simulink model "PubIfDecisionTOS_MDL"  (R2020b)
settings: configuration reference "DspaceConfig" (kept outside this file)
PostLoadFcn:
  | if any(exist('dsrtsu_mdlpostloadfcn', 'file') ~= 0), dsrtsu_mdlpostloadfcn('Execute', bdroot); end
InitFcn:
  | , if any(exist('dsmpb_private', 'file') ~= 0), dsmpb_private('dsmpb_mdlclblib', 'Init', bdroot); end,
undefined symbols (not defined in the file or in its folder): C_TOS_ACCEgoRAxletoFbumplength_m, C_TOS_ACCTargetFront_Flag, C_TOS_AEBJAPedObjDxThre_Val, C_TOS_AEBJAPedObjDyThre_Val, C_TOS_AEBJATargetSize_Val, C_TOS_AEBJAVehObjDxThre_Val, C_TOS_AEBJAVehObjDyThre_Val, C_TOS_AEBJuncPedTargetSize_Val, C_TOS_AEBLatObjDxThre_Val, C_TOS_AEBLatPedDyThre_Val, C_TOS_AEBLatTargetSize_Val, C_TOS_AEBLongTargetInEgoFront_Flag, C_TOS_axAbsGround_Parameter, C_TOS_CameraConfirmedFlag, C_TOS_CNsubjWidth, C_TOS_CurrentLaneCoreMinWidth_Val, C_TOS_CutInProb_Val_Zero, C_TOS_CutOutProb_Val_Zero, C_TOS_D2R_Val, C_TOS_DefaultValueObjectToCenterLine_dy, C_TOS_EgoCarWidth_Val, C_TOS_EgoDxRefPoint_m, C_TOS_EgoRAxletoFbumplength_m, C_TOS_HalfWidthVehicle_Con, C_TOS_HWA_CurrentLaneFlag, C_TOS_HWA_LeftLaneFlag, C_TOS_HWA_MovingDir_Vaild, C_TOS_HWA_MovState_Vaild, C_TOS_HWA_RightLaneFlag, C_TOS_LaneLineCourseErrorFront, C_TOS_LaneLineCourseErrorRear, C_TOS_MotorbikeDefaultWidth_m, C_TOS_NumberOfEffectiveTargets, C_TOS_Obj_Age_Val, C_TOS_Objdx_Constraint_Val, C_TOS_ObjectDefaultWidth_m, C_TOS_ObjInCurrentLane_Val, C_TOS_ObjInCurrentLaneValid, C_TOS_ObjInLeftLaneValid, C_TOS_ObjInRightLaneValid, C_TOS_ObjNotInCurrentLane_Val, C_TOS_ObjNotREElementType, C_TOS_ObjPredictDis_dy_ConstantVal_Zeros, C_TOS_ObjToCenterLine_ConstantVal_Zeros, C_TOS_OFMObjIDInvilad_Val, C_TOS_PIL_LatDisCons_Val_zero, C_TOS_PIL_ObjectCutInFlag_b, C_TOS_PIL_ObjectCutOutFlag_b, C_TOS_PIL_ObjLaneProb_al_Val, C_TOS_PP_ObjFusType_FC_Confirm_b, C_TOS_PP_ObjFusType_FC_FR_Confirm_b, C_TOS_PP_ObjFusType_FR_Confirm_b, C_TOS_RE_80BoolDefault_Val, C_TOS_RE_80Single181Default_Val, C_TOS_RE_80Single255Default_Val, C_TOS_RE_80Uint8Default_Val, C_TOS_RE_D2R, C_TOS_RE_D_180_Val, C_TOS_RE_InvalidObjectID_Val, C_TOS_RE_InvalidTargetChainDir_Val ... (+142)
libraries: simulink x1650, TOS_LIB x361, canfdmsglib x14
(part 21 of 69)

== system PubIfDecisionTOS_MDL/TOS_20201112/TOS_2012080320/TOS/AEB/TOS_AEBLatCro_20201208/AEBLat_Object_Condition/AEBLat_TargetCondition ==
  Object_ID : Inport  OutDataTypeStr=uint8  Partition=on  PartitionDimension=1  PartitionWidth=1  PartitionOffset=0
  PP_ObjFusType_FC_FR_Confirm : Inport  Port=2  Partition=on  PartitionDimension=1  PartitionWidth=1  PartitionOffset=0
  PP_ObjFusType_FR_Confirm : Inport  Port=3  Partition=on  PartitionDimension=1  PartitionWidth=1  PartitionOffset=0
  ObjectType : Inport  Port=4  Partition=on  PartitionDimension=1  PartitionWidth=1  PartitionOffset=0
  Object_Dx : Inport  Port=5  Partition=on  PartitionDimension=1  PartitionWidth=1  PartitionOffset=0
  Object_Dy : Inport  Port=6  Partition=on  PartitionDimension=1  PartitionWidth=1  PartitionOffset=0
  PP_ObjMovingDirSignalProcessing : Inport  Port=7  Partition=on  PartitionDimension=1  PartitionWidth=1  PartitionOffset=0
  Object_HeadingAngle : Inport  Port=8  Partition=on  PartitionDimension=1  PartitionWidth=1  PartitionOffset=0
  Object_VX : Inport  Port=9  Partition=on  PartitionDimension=1  PartitionWidth=1  PartitionOffset=0
  Object_VY : Inport  Port=10  Partition=on  PartitionDimension=1  PartitionWidth=1  PartitionOffset=0
  VIE_EgoVelocity : Inport  Port=11
  psiDtOpt : Inport  Port=12
  AEBLat_Target_ObjectID_K1 : Inport  Port=13
  Compare To Constant : simulink/Logic and Bit Operations/Compare To Constant  relop===  const=C_TOS_OFMObjIDInvilad_Val  OutDataTypeStr=boolean
      settings: AttributesFormatString=C_TOS_OFMObjIDInvilad_Val = 0
  For Each : ForEach  DisableCoverage=on
  If : If  IfExpression=u1 ~= 0
  Merge{,1..4} (5 alike) : Merge
  TOS_AEBLat_TargetsDx : Subsystem
  TOS_AEBLat_TargetsDxDefault : Subsystem  TreatAsAtomicUnit=on
  TOS_AEBLat_Targets_Dx : Outport  ConcatenationDimension=1
  AEBLat_TargetFusionType_observal : Outport  Port=2  ConcatenationDimension=1
  AEBLat_TargetObjectType_observal : Outport  Port=3  ConcatenationDimension=1
  AEBLat_TargetDXDY_observal : Outport  Port=4  ConcatenationDimension=1
  AEBLat_TargetMovDir_observal : Outport  Port=5  ConcatenationDimension=1
  wires:
  PP_ObjFusType_FC_FR_Confirm/1 -> TOS_AEBLat_TargetsDx/2(PP_ObjFusType_FC_FR_Confirm)
  PP_ObjFusType_FR_Confirm/1 -> TOS_AEBLat_TargetsDx/3(PP_ObjFusType_FR_Confirm)
  Object_VY/1 -> TOS_AEBLat_TargetsDx/10(Object_VY)
  VIE_EgoVelocity/1 -> TOS_AEBLat_TargetsDx/11(VIE_EgoVelocity)
  Object_VX/1 -> TOS_AEBLat_TargetsDx/9(Object_VX)
  PP_ObjMovingDirSignalProcessing/1 -> TOS_AEBLat_TargetsDx/7(PP_ObjMovingDirSignalProcessing)
  Object_HeadingAngle/1 -> TOS_AEBLat_TargetsDx/8(Object_HeadingAngle)
  ObjectType/1 -> TOS_AEBLat_TargetsDx/4(ObjectType)
  TOS_AEBLat_TargetsDxDefault/1(TOS_AEBLong_TargetsDx) -> Merge/1
  If/2 -> TOS_AEBLat_TargetsDx/Action
  If/1 -> TOS_AEBLat_TargetsDxDefault/Action
  Object_ID/1 -> Compare To Constant/1, [Object_ID]
  Compare To Constant/1 -> If/1
  TOS_AEBLat_TargetsDx/1(TOS_AEBLat_TargetsDx) -> Merge/2
  Object_Dy/1 -> TOS_AEBLat_TargetsDx/6(Object_Dy)
  Object_Dx/1 -> TOS_AEBLat_TargetsDx/5(Object_Dx)
  Merge/1 -> TOS_AEBLat_Targets_Dx/1
  TOS_AEBLat_TargetsDx/2(AEBLat_TargetFusionType_observal) -> Merge1/2
  TOS_AEBLat_TargetsDxDefault/2(AEBLong_TargetFusionType_observal) -> Merge1/1
  TOS_AEBLat_TargetsDxDefault/3(AEBLong_TargetObjectType_observal) -> Merge2/1
  TOS_AEBLat_TargetsDx/3(AEBLat_TargetObjectType_observal) -> Merge2/2
  TOS_AEBLat_TargetsDx/4(AEBLat_TargetDXDY_observal) -> Merge3/2
  TOS_AEBLat_TargetsDxDefault/4(AEBLong_TargetDXDY_observal) -> Merge3/1
  TOS_AEBLat_TargetsDxDefault/5(AEBLong_TargetMovDir_observal) -> Merge4/1
  TOS_AEBLat_TargetsDx/5(AEBLat_TargetMovDir_observal) -> Merge4/2
  Merge1/1 -> AEBLat_TargetFusionType_observal/1
  Merge2/1 -> AEBLat_TargetObjectType_observal/1
  Merge3/1 -> AEBLat_TargetDXDY_observal/1
  Merge4/1 -> AEBLat_TargetMovDir_observal/1
  [Object_ID] -> TOS_AEBLat_TargetsDx/1(Object_ID)  "Object_ID"
  AEBLat_Target_ObjectID_K1/1 -> TOS_AEBLat_TargetsDx/13(AEBLat_Target_ObjectID_K1)
  psiDtOpt/1 -> TOS_AEBLat_TargetsDx/12(psiDtOpt)

== system PubIfDecisionTOS_MDL/TOS_20201112/TOS_2012080320/TOS/AEB/TOS_AEBLatCro_20201208/AEBLat_Object_Condition2/AEBLat_TargetCondition ==
  Object_ID : Inport  OutDataTypeStr=uint8  Partition=on  PartitionDimension=1  PartitionWidth=1  PartitionOffset=0
  PP_ObjFusType_FC_FR_Confirm : Inport  Port=2  Partition=on  PartitionDimension=1  PartitionWidth=1  PartitionOffset=0
  PP_ObjFusType_FR_Confirm : Inport  Port=3  Partition=on  PartitionDimension=1  PartitionWidth=1  PartitionOffset=0
  ObjectType : Inport  Port=4  Partition=on  PartitionDimension=1  PartitionWidth=1  PartitionOffset=0
  Object_Dx : Inport  Port=5  Partition=on  PartitionDimension=1  PartitionWidth=1  PartitionOffset=0
  Object_Dy : Inport  Port=6  Partition=on  PartitionDimension=1  PartitionWidth=1  PartitionOffset=0
  PP_ObjMovingDirSignalProcessing : Inport  Port=7  Partition=on  PartitionDimension=1  PartitionWidth=1  PartitionOffset=0
  Object_HeadingAngle : Inport  Port=8  Partition=on  PartitionDimension=1  PartitionWidth=1  PartitionOffset=0
  Object_VX : Inport  Port=9  Partition=on  PartitionDimension=1  PartitionWidth=1  PartitionOffset=0
  Object_VY : Inport  Port=10  Partition=on  PartitionDimension=1  PartitionWidth=1  PartitionOffset=0
  VIE_EgoVelocity : Inport  Port=11
  psiDtOpt : Inport  Port=12
  AEBLat_Target_ObjectID_K1 : Inport  Port=13
  Compare To Constant : simulink/Logic and Bit Operations/Compare To Constant  relop===  const=C_TOS_OFMObjIDInvilad_Val  OutDataTypeStr=boolean
      settings: AttributesFormatString=C_TOS_OFMObjIDInvilad_Val = 0
  For Each : ForEach  DisableCoverage=on
  If : If  IfExpression=u1 ~= 0
  Merge{,1..4} (5 alike) : Merge
  TOS_AEBLat_TargetsDx : Subsystem
  TOS_AEBLat_TargetsDxDefault : Subsystem  TreatAsAtomicUnit=on
  TOS_AEBLat_Targets_Dx : Outport  ConcatenationDimension=1
  AEBLat_TargetFusionType_observal : Outport  Port=2  ConcatenationDimension=1
  AEBLat_TargetObjectType_observal : Outport  Port=3  ConcatenationDimension=1
  AEBLat_TargetDXDY_observal : Outport  Port=4  ConcatenationDimension=1
  AEBLat_TargetMovDir_observal : Outport  Port=5  ConcatenationDimension=1
  wires:
  PP_ObjFusType_FC_FR_Confirm/1 -> TOS_AEBLat_TargetsDx/2(PP_ObjFusType_FC_FR_Confirm)
  PP_ObjFusType_FR_Confirm/1 -> TOS_AEBLat_TargetsDx/3(PP_ObjFusType_FR_Confirm)
  Object_VY/1 -> TOS_AEBLat_TargetsDx/10(Object_VY)
  VIE_EgoVelocity/1 -> TOS_AEBLat_TargetsDx/11(VIE_EgoVelocity)
  Object_VX/1 -> TOS_AEBLat_TargetsDx/9(Object_VX)
  PP_ObjMovingDirSignalProcessing/1 -> TOS_AEBLat_TargetsDx/7(PP_ObjMovingDirSignalProcessing)
  Object_HeadingAngle/1 -> TOS_AEBLat_TargetsDx/8(Object_HeadingAngle)
  ObjectType/1 -> TOS_AEBLat_TargetsDx/4(ObjectType)
  TOS_AEBLat_TargetsDxDefault/1(TOS_AEBLong_TargetsDx) -> Merge/1
  If/2 -> TOS_AEBLat_TargetsDx/Action
  If/1 -> TOS_AEBLat_TargetsDxDefault/Action
  Object_ID/1 -> Compare To Constant/1, [Object_ID]
  Compare To Constant/1 -> If/1
  TOS_AEBLat_TargetsDx/1(TOS_AEBLat_TargetsDx) -> Merge/2
  Object_Dy/1 -> TOS_AEBLat_TargetsDx/6(Object_Dy)
  Object_Dx/1 -> TOS_AEBLat_TargetsDx/5(Object_Dx)
  Merge/1 -> TOS_AEBLat_Targets_Dx/1
  TOS_AEBLat_TargetsDx/2(AEBLat_TargetFusionType_observal) -> Merge1/2
  TOS_AEBLat_TargetsDxDefault/2(AEBLong_TargetFusionType_observal) -> Merge1/1
  TOS_AEBLat_TargetsDxDefault/3(AEBLong_TargetObjectType_observal) -> Merge2/1
  TOS_AEBLat_TargetsDx/3(AEBLat_TargetObjectType_observal) -> Merge2/2
  TOS_AEBLat_TargetsDx/4(AEBLat_TargetDXDY_observal) -> Merge3/2
  TOS_AEBLat_TargetsDxDefault/4(AEBLong_TargetDXDY_observal) -> Merge3/1
  TOS_AEBLat_TargetsDxDefault/5(AEBLong_TargetMovDir_observal) -> Merge4/1
  TOS_AEBLat_TargetsDx/5(AEBLat_TargetMovDir_observal) -> Merge4/2
  Merge1/1 -> AEBLat_TargetFusionType_observal/1
  Merge2/1 -> AEBLat_TargetObjectType_observal/1
  Merge3/1 -> AEBLat_TargetDXDY_observal/1
  Merge4/1 -> AEBLat_TargetMovDir_observal/1
  [Object_ID] -> TOS_AEBLat_TargetsDx/1(Object_ID)  "Object_ID"
  AEBLat_Target_ObjectID_K1/1 -> TOS_AEBLat_TargetsDx/13(AEBLat_Target_ObjectID_K1)
  psiDtOpt/1 -> TOS_AEBLat_TargetsDx/12(psiDtOpt)

== system PubIfDecisionTOS_MDL/TOS_20201112/TOS_2012080320/TOS/AEB/TOS_AEBLong/AEBLongTargetInfor/AEBLongTargetMovingDir ==
  TOS_AddAttributes : Inport
  TOS_AEBLongTargetIndex : Inport  Port=2  OutDataTypeStr=uint8
  AEBLongTargetInfroDefault : Subsystem  TreatAsAtomicUnit=on
  AEBLongTargetMovingDir : Subsystem  TreatAsAtomicUnit=on
  Compare To Constant1 : simulink/Logic and Bit Operations/Compare To Constant  relop===  const=C_TOS_OFMObjIDInvilad_Val  OutDataTypeStr=boolean
      settings: AttributesFormatString=C_TOS_OFMObjIDInvilad_Val = 0
  If : If  IfExpression=u1
  Merge : Merge
  TOS_AEBLongTargetMovingDir : Outport
  wires:
  Merge/1 -> TOS_AEBLongTargetMovingDir/1
  AEBLongTargetInfroDefault/1(TOS_AEBLongTargetMovingDir) -> Merge/1
  AEBLongTargetMovingDir/1(TOS_AEBLongTargetMovingDir) -> Merge/2
  If/2 -> AEBLongTargetMovingDir/Action
  If/1 -> AEBLongTargetInfroDefault/Action
  TOS_AddAttributes/1 -> AEBLongTargetMovingDir/1(TOS_AddAttributes)
  Compare To Constant1/1 -> If/1
  TOS_AEBLongTargetIndex/1 -> Compare To Constant1/1, AEBLongTargetMovingDir/2(TOS_AEBLongTargetIndex)

== system PubIfDecisionTOS_MDL/TOS_20201112/TOS_2012080320/TOS/AEB/TOS_AEBLong/AEBLong_Confirm/AEBLong ==
  Object_ID : Inport
  AEBLong_Index : Inport  Port=2
  Object_DX : Inport  Port=3
  Object_ObstacleProb : Inport  Port=4
  Object_ExistProb : Inport  Port=5
  Object_Fus_Type : Inport  Port=6
  object_MovingState : Inport  Port=7
  Object_HeadingAngle : Inport  Port=8
  Object_Type : Inport  Port=9
  VIE_EgoVelocity : Inport  Port=10
  PIL_LeftLaneProb : Inport  Port=11
  PIL_CurrentLaneProb : Inport  Port=12
  PIL_RightLaneProb : Inport  Port=13
  PP_MovingStateSignalProcessing : Inport  Port=14
  PP_ObjMovingDirSignalProcessing : Inport  Port=15
  PP_ObjectToCenterLine_dy : Inport  Port=16
  TLJ_TargetInCLValidityflg : Inport  Port=17
  PP_CurrentLaneWidth : Inport  Port=18
  Object_DY : Inport  Port=19
  SteerWheelAng : Inport  Port=20
  SteerWheelSpd : Inport  Port=21
  PP_ObjFusType_FC_FR_Confirm : Inport  Port=22
  PP_ObjFusType_FR_Confirm : Inport  Port=23
  PP_ObjFusType_FC_Confirm : Inport  Port=24
  Object_VX : Inport  Port=25
  Object_VY : Inport  Port=26
  PIL_OverlapRatio : Inport  Port=27
  AEBLong_Target_ID_K1 : Inport  Port=28
  AEBLong_Target_ID_K2 : Inport  Port=29
  AEBLong_Target_MovState_K1 : Inport  Port=30
  AEBLong_Target_MovState_K2 : Inport  Port=31
  AEBLong_TrgConfirm : Subsystem
  AEBLong_TrgConfirmDefault : Subsystem  TreatAsAtomicUnit=on
  Compare To Constant : simulink/Logic and Bit Operations/Compare To Constant  relop===  const=C_TOS_OFMObjIDInvilad_Val  OutDataTypeStr=boolean
      settings: AttributesFormatString=C_TOS_OFMObjIDInvilad_Val = 0
  Constant : Constant  Value=0  OutDataTypeStr=uint8
  If : If  IfExpression=u1 ~= 0
  Merge{,1..10} (11 alike) : Merge
  Switch : Switch  Criteria=u2 > Threshold
  TOS_AEBLong_TargetIndex : Outport
  TOS_AEBLong_TargetDis_ObserVale : Outport  Port=2
  TOS_AEBLong_ObstacleProb_ObserVale : Outport  Port=3
  TOS_AEBLong_TargetExistProb_ObserVale : Outport  Port=4
  TOS_AEBLong_ObjFusType_ObserVale : Outport  Port=5
  TOS_AEBLong_TargetInEgoFront_ObserVale : Outport  Port=6
  TOS_AEBLong_TargetMovingDir_ObserVale : Outport  Port=7
  TOS_AEB_Stockade_ObserVale : Outport  Port=8
  TOS_AEBLong_TargetDy_ObserVale : Outport  Port=9
  TOS_AEBLong_SteerWheelAngConfirm_ObserVale : Outport  Port=10
  TOS_AEBLong_OverlapRatio_ObserVale : Outport  Port=11
  wires:
  AEBLong_Index/1 -> [AEBLong_Index], Compare To Constant/1
  Merge/1 -> Switch/2
  Compare To Constant/1 -> If/1
  If/1 -> AEBLong_TrgConfirmDefault/Action
  AEBLong_TrgConfirmDefault/1(TOS_AEBLong_TargetConditionJudge) -> Merge/1
  Object_ID/1 -> AEBLong_TrgConfirm/2(Object_ID)
  Object_DX/1 -> AEBLong_TrgConfirm/3(Object_DX)
  Object_ObstacleProb/1 -> AEBLong_TrgConfirm/4(Object_ObstacleProb)
  Object_ExistProb/1 -> AEBLong_TrgConfirm/5(Object_ExistProb)
  Object_Fus_Type/1 -> AEBLong_TrgConfirm/6(Object_Fus_Type)
  object_MovingState/1 -> AEBLong_TrgConfirm/7(object_MovingState)
  Object_HeadingAngle/1 -> AEBLong_TrgConfirm/8(Object_HeadingAngle)
  Object_Type/1 -> AEBLong_TrgConfirm/9(Object_Type)
  VIE_EgoVelocity/1 -> AEBLong_TrgConfirm/10(VIE_EgoVelocity)
  PIL_LeftLaneProb/1 -> AEBLong_TrgConfirm/11(PIL_LeftLaneProb)
  PIL_CurrentLaneProb/1 -> AEBLong_TrgConfirm/12(PIL_CurrentLaneProb)
  PIL_RightLaneProb/1 -> AEBLong_TrgConfirm/13(PIL_RightLaneProb)
  PP_MovingStateSignalProcessing/1 -> AEBLong_TrgConfirm/14(PP_MovingStateSignalProcessing)
  PP_ObjMovingDirSignalProcessing/1 -> AEBLong_TrgConfirm/15(PP_ObjMovingDirSignalProcessing)
  PP_ObjectToCenterLine_dy/1 -> AEBLong_TrgConfirm/16(PP_ObjectToCenterLine_dy)
  TLJ_TargetInCLValidityflg/1 -> AEBLong_TrgConfirm/17(TLJ_TargetInCLValidityflg)
  PP_CurrentLaneWidth/1 -> AEBLong_TrgConfirm/18(PP_CurrentLaneWidth)
  Object_DY/1 -> AEBLong_TrgConfirm/19(Object_DY)
  SteerWheelAng/1 -> AEBLong_TrgConfirm/20(SteerWheelAng)  "SteerWheelAng"
  SteerWheelSpd/1 -> AEBLong_TrgConfirm/21(SteerWheelSpd)  "SteerWheelSpd"
  AEBLong_TrgConfirm/1(TOS_AEBLong_TargetConditionJudge) -> Merge/2
  If/2 -> AEBLong_TrgConfirm/Action
  [AEBLong_Index] -> AEBLong_TrgConfirm/1(In1)
  [AEBLong_Index] -> Switch/1
  Switch/1 -> TOS_AEBLong_TargetIndex/1
  Constant/1 -> Switch/3
  Merge7/1 -> TOS_AEBLong_TargetMovingDir_ObserVale/1
  Merge3/1 -> TOS_AEBLong_ObstacleProb_ObserVale/1
  Merge8/1 -> TOS_AEB_Stockade_ObserVale/1
  Merge10/1 -> TOS_AEBLong_SteerWheelAngConfirm_ObserVale/1
  Merge2/1 -> TOS_AEBLong_TargetDis_ObserVale/1
  Merge6/1 -> TOS_AEBLong_TargetInEgoFront_ObserVale/1
  Merge4/1 -> TOS_AEBLong_TargetExistProb_ObserVale/1
  Merge9/1 -> TOS_AEBLong_TargetDy_ObserVale/1
  Merge5/1 -> TOS_AEBLong_ObjFusType_ObserVale/1
  AEBLong_TrgConfirm/10(TOS_AEBLong_SteerWheelAngConfirm_ObserVale) -> Merge10/2
  AEBLong_TrgConfirm/2(TOS_AEBLong_TargetDis_ObserVale) -> Merge2/2
  AEBLong_TrgConfirm/3(TOS_AEBLong_ObstacleProb_ObserVale) -> Merge3/2
  AEBLong_TrgConfirm/4(TOS_AEBLong_TargetExistProb_ObserVale) -> Merge4/2
  AEBLong_TrgConfirm/5(TOS_AEBLong_ObjFusType_ObserVale) -> Merge5/2
  AEBLong_TrgConfirm/6(TOS_AEBLong_TargetInEgoFront_ObserVale) -> Merge6/2
  AEBLong_TrgConfirm/7(TOS_AEBLong_TargetMovingDir_ObserVale) -> Merge7/2
  AEBLong_TrgConfirm/8(TOS_AEB_Stockade_ObserVale) -> Merge8/2
  AEBLong_TrgConfirm/9(TOS_AEBLong_TargetDy_ObserVale) -> Merge9/2
  AEBLong_TrgConfirmDefault/2(TOS_AEBLong_TargetDis_ObserVale) -> Merge2/1
  AEBLong_TrgConfirmDefault/3(TOS_AEBLong_ObstacleProb_ObserVale) -> Merge3/1
  AEBLong_TrgConfirmDefault/4(TOS_AEBLong_TargetExistProb_ObserVale) -> Merge4/1
  AEBLong_TrgConfirmDefault/5(TOS_AEBLong_ObjFusType_ObserVale) -> Merge5/1
  AEBLong_TrgConfirmDefault/6(TOS_AEBLong_TargetInEgoFront_ObserVale) -> Merge6/1
  AEBLong_TrgConfirmDefault/7(TOS_AEBLong_TargetMovingDir_ObserVale) -> Merge7/1
  AEBLong_TrgConfirmDefault/8(TOS_AEB_Stockade_ObserVale) -> Merge8/1
  AEBLong_TrgConfirmDefault/9(TOS_AEBLong_TargetDy_ObserVale) -> Merge9/1
  AEBLong_TrgConfirmDefault/10(TOS_AEBLong_SteerWheelAngConfirm_ObserVale) -> Merge10/1
  PP_ObjFusType_FC_FR_Confirm/1 -> AEBLong_TrgConfirm/22(PP_ObjFusType_FC_FR_Confirm)
  PP_ObjFusType_FR_Confirm/1 -> AEBLong_TrgConfirm/23(PP_ObjFusType_FR_Confirm)
  PP_ObjFusType_FC_Confirm/1 -> AEBLong_TrgConfirm/24(PP_ObjFusType_FC_Confirm)
  Object_VX/1 -> AEBLong_TrgConfirm/25(Object_VX)
  Object_VY/1 -> AEBLong_TrgConfirm/26(Object_VY)
  PIL_OverlapRatio/1 -> AEBLong_TrgConfirm/27(PIL_OverlapRatio)
  AEBLong_TrgConfirmDefault/11(TOS_AEBLong_OverlapRatio_ObserVale) -> Merge1/1
  AEBLong_TrgConfirm/11(TOS_AEBLong_OverlapRatio_ObserVale) -> Merge1/2
  Merge1/1 -> TOS_AEBLong_OverlapRatio_ObserVale/1
  AEBLong_Target_ID_K1/1 -> AEBLong_TrgConfirm/28(AEBLong_Target_ID_K1)
  AEBLong_Target_ID_K2/1 -> AEBLong_TrgConfirm/29(AEBLong_Target_ID_K2)
  AEBLong_Target_MovState_K1/1 -> AEBLong_TrgConfirm/30(AEBLong_Target_MovState_K1)
  AEBLong_Target_MovState_K2/1 -> AEBLong_TrgConfirm/31(AEBLong_Target_MovState_K2)

== system PubIfDecisionTOS_MDL/TOS_20201112/TOS_2012080320/TOS/AEB/TOS_AEBLong/AEBLong_Confirm/TOS_AEBLong_ObserVale ==
  note: Obj_ID
  note: SteerWheelAngConfirm
  note: TargetDy
  note: Stockade
  note: TargetMovingDir
  note: TargetInEgoFront
  note: ObjFusType
  note: TargetExistProb
  note: ObstacleProb
  note: TargetDis
  TOS_AEBLong_TargetIndex : Inport
  TOS_AEBLong_ObserVale : Inport  Port=2
  Bus Selector3 : BusSelector  OutputSignals=TOS_AEBLong_TargetDis_ObserVale,TOS_AEBLong_ObstacleProb_ObserVale,TOS_AEBLong_TargetExistProb_ObserVale,TOS_AEBLong_ObjFusType_ObserVale,TOS_AEBLong_TargetInEgoFront_ObserVale,TOS_AEBLong_TargetMovingDir_ObserVale,TOS_AEB_Stockade_ObserVale,TOS_AEBLong_TargetDy_ObserVale,TOS_AEBLong_SteerWheelAngConfirm_ObserVale,TOS_AEBLong_OverlapRatio_ObserVale
  Display{,1..6,23..26} (11 alike) : Display
  wires:
  TOS_AEBLong_ObserVale/1 -> Bus Selector3/1
  Bus Selector3/1 -> [TOS_AEBLong_TargetDis_ObserVale]  "<TOS_AEBLong_TargetDis_ObserVale>"
  Bus Selector3/2 -> [TOS_AEBLong_ObstacleProb_ObserVale]  "<TOS_AEBLong_ObstacleProb_ObserVale>"
  Bus Selector3/3 -> [TOS_AEBLong_TargetExistProb_ObserVale]  "<TOS_AEBLong_TargetExistProb_ObserVale>"
  Bus Selector3/4 -> [TOS_AEBLong_ObjFusType_ObserVale]  "<TOS_AEBLong_ObjFusType_ObserVale>"
  Bus Selector3/5 -> [TOS_AEBLong_TargetInEgoFront_ObserVale]  "<TOS_AEBLong_TargetInEgoFront_ObserVale>"
  Bus Selector3/6 -> [TOS_AEBLong_TargetMovingDir_ObserVale]  "<TOS_AEBLong_TargetMovingDir_ObserVale>"
  Bus Selector3/7 -> [TOS_AEB_Stockade_ObserVale]  "<TOS_AEB_Stockade_ObserVale>"
  Bus Selector3/8 -> [TOS_AEB_TargetDy_ObserVale]  "<TOS_AEBLong_TargetDy_ObserVale>"
  Bus Selector3/9 -> [TOS_AEBLong_SteerWheelAngConfirm_ObserVale]  "<TOS_AEBLong_SteerWheelAngConfirm_ObserVale>"
  [TOS_AEBLong_TargetDis_ObserVale] -> Display26/1
  [TOS_AEBLong_ObstacleProb_ObserVale] -> Display25/1
  [TOS_AEBLong_TargetExistProb_ObserVale] -> Display24/1
  [TOS_AEBLong_ObjFusType_ObserVale] -> Display23/1
  [TOS_AEBLong_TargetInEgoFront_ObserVale] -> Display/1
  [TOS_AEBLong_TargetMovingDir_ObserVale] -> Display1/1
  [TOS_AEB_Stockade_ObserVale] -> Display2/1
  [TOS_AEB_TargetDy_ObserVale] -> Display3/1
  [TOS_AEBLong_SteerWheelAngConfirm_ObserVale] -> Display4/1
  TOS_AEBLong_TargetIndex/1 -> Display5/1
  Bus Selector3/10 -> [TOS_AEBLong_OverlapRatio_ObserVale]  "<TOS_AEBLong_OverlapRatio_ObserVale>"
  [TOS_AEBLong_OverlapRatio_ObserVale] -> Display6/1

== system PubIfDecisionTOS_MDL/TOS_20201112/TOS_2012080320/TOS/AEB/TOS_AEBLong/AEBLong_Target_PreJudge/AEBLONG_Target_PreFilt ==
  PP_ObjFusType_FC_FR_Confirm : Inport  Partition=on  PartitionDimension=1  PartitionWidth=1  PartitionOffset=0
  PP_ObjFusType_FR_Confirm : Inport  Port=2  Partition=on  PartitionDimension=1  PartitionWidth=1  PartitionOffset=0
  PP_ObjFusType_FC_Confirm : Inport  Port=3  Partition=on  PartitionDimension=1  PartitionWidth=1  PartitionOffset=0
  Object_ID : Inport  Port=4  OutDataTypeStr=uint8  Partition=on  PartitionDimension=1  PartitionWidth=1  PartitionOffset=0
  Obj_MovingState : Inport  Port=5  Partition=on  PartitionDimension=1  PartitionWidth=1  PartitionOffset=0
  Obj_Dx : Inport  Port=6  Partition=on  PartitionDimension=1  PartitionWidth=1  PartitionOffset=0
  Object_ObstacleProb : Inport  Port=7  Partition=on  PartitionDimension=1  PartitionWidth=1  PartitionOffset=0
  Object_DY : Inport  Port=8  Partition=on  PartitionDimension=1  PartitionWidth=1  PartitionOffset=0
  AEBLONG_Target_ID_K1 : Inport  Port=9
  AEBLONG_Target_Dx_K1 : Inport  Port=10
  PP_REElementType : Inport  Port=11  Partition=on  PartitionDimension=1  PartitionWidth=1  PartitionOffset=0
  AEBLONG_TargetPreCondJudge : Subsystem
  AEBLONG_TargetPreCondJudgeDefault : Subsystem  TreatAsAtomicUnit=on
  Compare To Constant : simulink/Logic and Bit Operations/Compare To Constant  relop===  const=C_TOS_OFMObjIDInvilad_Val  OutDataTypeStr=boolean
      settings: AttributesFormatString=C_TOS_OFMObjIDInvilad_Val = 0
  For Each : ForEach  DisableCoverage=on
  If : If  IfExpression=u1 ~= 0
  Merge{,1..4} (5 alike) : Merge
  TOS_AEBLONG_Target_PreFiltFlag : Outport  ConcatenationDimension=1
  TOS_AEBLONG_Target_FusionTypeFlag_ObserVale : Outport  Port=2  ConcatenationDimension=1
  TOS_AEBLONG_Target_PassedbyTarget_Flag_ObserVale : Outport  Port=3  ConcatenationDimension=1
  TOS_AEBLONG_Target_FenceFlag_ObserVale : Outport  Port=4  ConcatenationDimension=1
  TOS_AEBLONG_Target_REElementType_ObserVale : Outport  Port=5  ConcatenationDimension=1
  wires:
  Merge/1 -> TOS_AEBLONG_Target_PreFiltFlag/1
  PP_ObjFusType_FC_FR_Confirm/1 -> AEBLONG_TargetPreCondJudge/2(PP_ObjFusType_FC_FR_Confirm)
  PP_ObjFusType_FR_Confirm/1 -> AEBLONG_TargetPreCondJudge/3(PP_ObjFusType_FR_Confirm)
  AEBLONG_TargetPreCondJudge/1(TOS_AEBLONG_Target_PreFiltFlag) -> Merge/2
  Compare To Constant/1 -> If/1
  Object_ID/1 -> [Object_ID], Compare To Constant/1
  If/1 -> AEBLONG_TargetPreCondJudgeDefault/Action
  If/2 -> AEBLONG_TargetPreCondJudge/Action
  AEBLONG_TargetPreCondJudgeDefault/1(TOS_AEBLONG_Target_PreFiltFlag) -> Merge/1
  PP_ObjFusType_FC_Confirm/1 -> AEBLONG_TargetPreCondJudge/4(PP_ObjFusType_FC_Confirm)
  Obj_MovingState/1 -> AEBLONG_TargetPreCondJudge/5(Obj_MovingState)  "Obj_MovingState"
  Obj_Dx/1 -> AEBLONG_TargetPreCondJudge/6(Obj_Dx)  "Obj_Dx"
  Object_ObstacleProb/1 -> AEBLONG_TargetPreCondJudge/7(Object_ObstacleProb)  "Object_ObstacleProb"
  Object_DY/1 -> AEBLONG_TargetPreCondJudge/8(Object_DY)  "Object_DY"
  [Object_ID] -> AEBLONG_TargetPreCondJudge/1(Object_ID)
  AEBLONG_TargetPreCondJudge/2(TOS_AEBLONG_Target_FusionTypeFlag_ObserVale) -> Merge1/2
  AEBLONG_TargetPreCondJudge/3(TOS_AEBLONG_Target_PassedbyTarget_Flag_ObserVale) -> Merge2/2
  AEBLONG_TargetPreCondJudge/4(TOS_AEBLONG_Target_FenceFlag_ObserVale) -> Merge3/2
  AEBLONG_TargetPreCondJudgeDefault/2(TOS_AEBLONG_Target_FusionTypeFlag_ObserVale) -> Merge1/1
  AEBLONG_TargetPreCondJudgeDefault/3(TOS_AEBLONG_Target_PassedbyTarget_Flag_ObserVale) -> Merge2/1
  AEBLONG_TargetPreCondJudgeDefault/4(TOS_AEBLONG_Target_FenceFlag_ObserVale) -> Merge3/1
  Merge1/1 -> TOS_AEBLONG_Target_FusionTypeFlag_ObserVale/1
  Merge2/1 -> TOS_AEBLONG_Target_PassedbyTarget_Flag_ObserVale/1
  Merge3/1 -> TOS_AEBLONG_Target_FenceFlag_ObserVale/1
  AEBLONG_Target_ID_K1/1 -> AEBLONG_TargetPreCondJudge/9(AEBLONG_Target_ID_K1)  "AEBLONG_Target_ID_K1"
  AEBLONG_Target_Dx_K1/1 -> AEBLONG_TargetPreCondJudge/10(AEBLONG_Target_Dx_K1)  "AEBLONG_Target_Dx_K1"
  PP_REElementType/1 -> AEBLONG_TargetPreCondJudge/11(PP_REElementType)  "PP_REElementType"
  AEBLONG_TargetPreCondJudge/5(TOS_AEBLONG_Target_REElementType_ObserVale) -> Merge4/2
  AEBLONG_TargetPreCondJudgeDefault/5(TOS_AEBLONG_Target_REElementType_ObserVale) -> Merge4/1
  Merge4/1 -> TOS_AEBLONG_Target_REElementType_ObserVale/1

== system PubIfDecisionTOS_MDL/TOS_20201112/TOS_2012080320/TOS/LC_LCKie_ELK/TOS_HWA/CurrentLane/HWA_CurrentLane_Target ==
  note: 本车道前方，最近目标
  note: 前方次近
  VIE_EgoVelocity : Inport
  OFM_SignalVerification : Inport  Port=2
  TOS_AddAttributes : Inport  Port=3
  TOS_TLJ_SameLaneConfirm_Flag : Inport  Port=4
  TOS_ProbInLaneCalculat : Inport  Port=5
  TOS_VCAN_SignalVerification : Inport  Port=6
  LM_LR_Line04_dDisStart : Inport  Port=7
  LM_LR_Line04_dDisEnd : Inport  Port=8
  LM_LR_Line05_dDisStart : Inport  Port=9
  LM_LR_Line05_dDisEnd : Inport  Port=10
  LM_LR_Line06_dDisStart : Inport  Port=11
  LM_LR_Line06_dDisEnd : Inport  Port=12
  LM_LR_Line04_pC2 : Inport  Port=13
  LM_LR_Line05_pC2 : Inport  Port=14
  LM_LR_Line06_pC2 : Inport  Port=15
  LM_LR_Line04_fCamValid : Inport  Port=16
  LM_LR_Line05_fCamValid : Inport  Port=17
  LM_LR_Line06_fCamValid : Inport  Port=18
  LM_LR_Line04_pC0 : Inport  Port=19
  LM_RL_Line04_pC0 : Inport  Port=20
  TOS_HWA_Target_ID_K1 : Inport  Port=21
  TOS_HWA_Target_MovState_K1 : Inport  Port=22
  TOS_HWA_CurrentLane_ObjIndex : Inport  Port=23
  Bus Creator : BusCreator  Inputs=29
  Bus Creator1 : BusCreator  Inputs=18
  Bus Creator2 : BusCreator  Inputs=18
  Bus Creator3 : BusCreator  Inputs=5
  Bus Selector : BusSelector  OutputSignals=TOS_HWA_CurrentLane_ObjIndex,OFM_SignalVerification.Object_ID,OFM_SignalVerification.Object_Fus_Type,OFM_SignalVerification.Object_MovingState,TOS_AddAttributes.PP_ObjMovingDirSignalProcessing,OFM_SignalVerification.Object_HeadingAngle,OFM_SignalVerification.Object_DX,TOS_TLJ_SameLaneConfirm_Flag,OFM_SignalVerification.Object_Type,OFM_SignalVerification.Object_ObstacleProb,OFM_SignalVerification.Object_DY,TOS_AddAttributes.PP_ObjFusType_FC_FR_Confirm,TOS_AddAttributes.PP_ObjFusType_FR_Confirm,TOS_AddAttributes.PP_ObjFusType_FC_Confirm,OFM_SignalVerification.Object_VX,OFM_SignalVerification.Object_VY,VIE_EgoVelocity,TOS_VCAN_SignalVerification.SteerWheelAng,TOS_ProbInLaneCalculat.PIL_OverlapRatio,HWA_CLF_Target_2_ID_K1,HWA_CLF_Target_2_ID_K2,HWA_CLF_Target_2_MovState_K1,HWA_CLF_Target_2_MovState_K2,LM_LR_Line04_dDisStart,LM_LR_Line04_dDisEnd,LM_LR_Line05_dDisStart,LM_LR_Line05_dDisEnd,LM_LR_Line06_dDisStart,LM_LR_Line06_dDisEnd,LM_LR_Line04_pC2,LM_LR_Line05_pC2,LM_LR_Line06_pC2,LM_LR_Line04_fCamValid,LM_LR_Line05_fCamValid,LM_LR_Line06_fCamValid,LM_LR_Line04_pC0,LM_RL_Line04_pC0
  Bus Selector1 : BusSelector  OutputSignals=TOS_HWA_CurrentLane_ObjIndex,OFM_SignalVerification.Object_ID,OFM_SignalVerification.Object_Fus_Type,OFM_SignalVerification.Object_MovingState,TOS_AddAttributes.PP_ObjMovingDirSignalProcessing,OFM_SignalVerification.Object_HeadingAngle,OFM_SignalVerification.Object_DX,TOS_TLJ_SameLaneConfirm_Flag,OFM_SignalVerification.Object_Type,OFM_SignalVerification.Object_ObstacleProb,OFM_SignalVerification.Object_DY,TOS_AddAttributes.PP_ObjFusType_FC_FR_Confirm,TOS_AddAttributes.PP_ObjFusType_FR_Confirm,TOS_AddAttributes.PP_ObjFusType_FC_Confirm,OFM_SignalVerification.Object_VX,OFM_SignalVerification.Object_VY,VIE_EgoVelocity,TOS_VCAN_SignalVerification.SteerWheelAng,TOS_ProbInLaneCalculat.PIL_OverlapRatio,HWA_CLF_Target_1_ID_K1,HWA_CLF_Target_1_ID_K2,HWA_CLF_Target_1_MovState_K1,HWA_CLF_Target_1_MovState_K2,LM_LR_Line04_dDisStart,LM_LR_Line04_dDisEnd,LM_LR_Line05_dDisStart,LM_LR_Line05_dDisEnd,LM_LR_Line06_dDisStart,LM_LR_Line06_dDisEnd,LM_LR_Line04_pC2,LM_LR_Line05_pC2,LM_LR_Line06_pC2,LM_LR_Line04_fCamValid,LM_LR_Line05_fCamValid,LM_LR_Line06_fCamValid,LM_LR_Line04_pC0,LM_RL_Line04_pC0
  Bus Selector2 : BusSelector  OutputSignals=TOS_HWA_CurrentLane_ObjIndex,TOS_AddAttributes.PP_ObjMovingDirSignalProcessing,OFM_SignalVerification.Object_VX,OFM_SignalVerification.Object_VY,OFM_SignalVerification.Object_Type,OFM_SignalVerification.Object_MovingState,TOS_TLJ_SameLaneConfirm_Flag,OFM_SignalVerification.Object_DX,OFM_SignalVerification.Object_DY,OFM_SignalVerification.Object_Fus_Type,OFM_SignalVerification.Object_HeadingAngle,TOS_AddAttributes.PP_ObjFusType_FC_FR_Confirm,TOS_AddAttributes.PP_ObjFusType_FR_Confirm,TOS_AddAttributes.PP_ObjFusType_FC_Confirm,VIE_EgoVelocity
  Constant : Constant  Value=10  OutDataTypeStr=uint8
  Constant1 : Constant  Value=9  OutDataTypeStr=uint8
  Data Type Conversion{1..4} (4 alike) : DataTypeConversion  OutDataTypeStr=Enum: ObjectMovingState_E
  Delay{,3..4,7} (4 alike) : Delay  InitialCondition=0
  Delay{1..2,5..6} (4 alike) : Delay  DelayLength=1  InitialCondition=0
  HWA_CLF_Target_1 : Subsystem
  HWA_CLF_Target_2 : Subsystem
  HWA_CLF_Target_3 : Subsystem
  Selector{1..4} (4 alike) : Selector  InputPortWidth=11  IndexOptions=Index vector (port)  Indices=[1 3]  OutputSizes=1
  Subsystem : Subsystem
  TOS_HWA_Target_ID_K2 : InportShadow  Port=21
  TOS_HWA_Target_MovState_K2 : InportShadow  Port=22
  Terminator : Terminator
  Terminator1 : Terminator
  Terminator2 : Terminator
  HWA_CLF_Target_1_Index : Outport
  HWA_CLF_Target_2_Index : Outport  Port=2
  HWA_CLR_Target_3_Index : Outport  Port=3
  TargetInCurrentLane_b : Outport  Port=4
  wires:
  TOS_TLJ_SameLaneConfirm_Flag/1 -> Bus Creator/4  "TOS_TLJ_SameLaneConfirm_Flag"
  TOS_AddAttributes/1 -> Bus Creator/3  "TOS_AddAttributes"
  OFM_SignalVerification/1 -> Bus Creator/2  "OFM_SignalVerification"
  VIE_EgoVelocity/1 -> Bus Creator/1  "VIE_EgoVelocity"
  TOS_ProbInLaneCalculat/1 -> Bus Creator/5  "TOS_ProbInLaneCalculat"
  Bus Selector/3 -> HWA_CLF_Target_2/3(Object_Fus_Type)  "<Object_Fus_Type>"
  Bus Selector/4 -> HWA_CLF_Target_2/4(object_MovingState)  "<Object_MovingState>"
  HWA_CLF_Target_2/1(HWA_CLF_Target_2_Index) -> [HWA_CLF_Target_2_Index], HWA_CLF_Target_2_Index/1  "HWA_CLF_Target_2_Index"
  Bus Selector/7 -> HWA_CLF_Target_2/7(Object_DX)  "<Object_DX>"
  Bus Selector/8 -> HWA_CLF_Target_2/8(TOS_TLJ_SameLaneConfirm_Flag)  "<TOS_TLJ_SameLaneConfirm_Flag>"
  Bus Selector/9 -> HWA_CLF_Target_2/9(Object_Type)  "<Object_Type>"
  Bus Selector/2 -> HWA_CLF_Target_2/2(Object_ID)  "<Object_ID>"
  HWA_CLF_Target_2/2(HWA_CLF_Target_FusionType_ObserVale) -> Bus Creator1/1  "HWA_CLF_Target_2_FusionType_ObserVale"
  HWA_CLF_Target_2/3(HWA_CLF_Target_TrgMovDir_ObserVale) -> Bus Creator1/2  "HWA_CLF_Target_2_TrgMovDir_ObserVale"
  HWA_CLF_Target_2/4(HWA_CLF_Target_TargetDxConfirm_ObserVale) -> Bus Creator1/3  "HWA_CLF_Target_2_TargetDxConfirm_ObserVale"
  HWA_CLF_Target_2/5(HWA_CLF_Target_ObjType_ObserVale) -> Bus Creator1/4  "HWA_CLF_Target_2_ObjType_ObserVale"
  Bus Selector/10 -> HWA_CLF_Target_2/10(Object_ObstacleProb)  "<Object_ObstacleProb>"
  HWA_CLF_Target_2/6(HWA_CLF_Target_ObstacleProb_ObserVale) -> Bus Creator1/5  "HWA_CLF_Target_2_ObstacleProb_ObserVale"
  Bus Selector/5 -> HWA_CLF_Target_2/5(PP_ObjMovingDirSignalProcessing)  "<PP_ObjMovingDirSignalProcessing>"
  Bus Selector/6 -> HWA_CLF_Target_2/6(Object_HeadingAngle)  "<Object_HeadingAngle>"
  Bus Selector/11 -> HWA_CLF_Target_2/11(Object_DY)  "<Object_DY>"
  HWA_CLF_Target_2/7(HWA_CLF_Target_DyConfirm_ObserVale) -> Bus Creator1/6  "HWA_CLF_Target_2_DyConfirm_ObserVale"
  Bus Creator1/1 -> Terminator/1  "HWA_CLF_Target_2_ObserVale"
  TOS_HWA_CurrentLane_ObjIndex/1 -> Bus Creator/21  "TOS_HWA_CurrentLane_ObjIndex"
  Bus Selector/1 -> HWA_CLF_Target_2/1(HWA_CLF_Trg_2_Index)  "<TOS_HWA_CurrentLane_ObjIndex>"
  Bus Selector/12 -> HWA_CLF_Target_2/12(PP_ObjFusType_FC_FR_Confirm)  "<PP_ObjFusType_FC_FR_Confirm>"
  Bus Selector/13 -> HWA_CLF_Target_2/13(PP_ObjFusType_FR_Confirm)  "<PP_ObjFusType_FR_Confirm>"
  Bus Selector/14 -> HWA_CLF_Target_2/14(PP_ObjFusType_FC_Confirm)  "<PP_ObjFusType_FC_Confirm>"
  Bus Selector/15 -> HWA_CLF_Target_2/15(Object_VX)  "<Object_VX>"
  Bus Selector/16 -> HWA_CLF_Target_2/16(Object_VY)  "<Object_VY>"
  Bus Selector/17 -> HWA_CLF_Target_2/17(VIE_EgoVelocity)  "<VIE_EgoVelocity>"
  TOS_VCAN_SignalVerification/1 -> Bus Creator/6  "TOS_VCAN_SignalVerification"
  Bus Selector/18 -> HWA_CLF_Target_2/18(SteerWheelAng)  "<SteerWheelAng>"
  Bus Selector/19 -> HWA_CLF_Target_2/19(PIL_OverlapRatio)  "<PIL_OverlapRatio>"
  HWA_CLF_Target_2/17(HWA_CLF_Target_DyConfirm_4_OverlapRatio_ObserVale) -> Bus Creator1/16  "HWA_CLF_Target_2_DyConfirm_4_OverlapRatio_ObserVale"
  Delay1/1 -> Bus Creator/22  "HWA_CLF_Target_2_ID_K1"
  Delay/1 -> Bus Creator/23  "HWA_CLF_Target_2_ID_K2"
  Delay2/1 -> Data Type Conversion2/1
  Data Type Conversion1/1 -> Bus Creator/25  "HWA_CLF_Target_2_MovState_K2"
  Bus Selector/20 -> HWA_CLF_Target_2/20(HWA_CLF_Target_ID_K1)  "<HWA_CLF_Target_2_ID_K1>"
  Bus Selector/21 -> HWA_CLF_Target_2/21(HWA_CLF_Target_ID_K2)  "<HWA_CLF_Target_2_ID_K2>"
  Bus Selector/22 -> HWA_CLF_Target_2/22(HWA_CLF_Target_MovState_K1)  "<HWA_CLF_Target_2_MovState_K1>"
  Bus Selector/23 -> HWA_CLF_Target_2/23(HWA_CLF_Target_MovState_K2)  "<HWA_CLF_Target_2_MovState_K2>"
  Selector2/1 -> Delay3/1, Delay2/1
  Data Type Conversion2/1 -> Bus Creator/24  "HWA_CLF_Target_2_MovState_K1"
  HWA_CLF_Target_2/8(HWA_CLF_Target_TrgMovDirFlag_1_ObserVale) -> Bus Creator1/7  "HWA_CLF_Target_2_TrgMovDirFlag_1_ObserVale"
  HWA_CLF_Target_2/9(HWA_CLF_Target_TrgMovDirFlag_2_ObserVale) -> Bus Creator1/8  "HWA_CLF_Target_2_TrgMovDirFlag_2_ObserVale"
  HWA_CLF_Target_2/10(HWA_CLF_Target_TrgMovDirFlag_3_ObserVale) -> Bus Creator1/9  "HWA_CLF_Target_2_TrgMovDirFlag_3_ObserVale"
  HWA_CLF_Target_2/11(HWA_CLF_Target_TrgMovDirFlag_4_ObserVale) -> Bus Creator1/10  "HWA_CLF_Target_2_TrgMovDirFlag_4_ObserVale"
  HWA_CLF_Target_2/12(HWA_CLF_Target_TrgMovDirFlag_5_ObserVale) -> Bus Creator1/11  "HWA_CLF_Target_2_TrgMovDirFlag_5_ObserVale"
  HWA_CLF_Target_2/14(HWA_CLF_Target_DyConfirm_1_ObserVale) -> Bus Creator1/13  "HWA_CLF_Target_2_DyConfirm_1_ObserVale"
  HWA_CLF_Target_2/15(HWA_CLF_Target_DyConfirm_2_ObserVale) -> Bus Creator1/14  "HWA_CLF_Target_2_DyConfirm_2_ObserVale"
  HWA_CLF_Target_2/16(HWA_CLF_Target_DyConfirm_3_ObserVale) -> Bus Creator1/15  "HWA_CLF_Target_2_DyConfirm_3_ObserVale"
  Delay3/1 -> Data Type Conversion1/1
  TOS_HWA_Target_ID_K1/1 -> Selector1/1
  Selector3/1 -> Delay4/1, Delay5/1
  Selector4/1 -> Delay7/1, Delay6/1
  Delay5/1 -> Bus Creator/26  "HWA_CLF_Target_1_ID_K1"
  Delay4/1 -> Bus Creator/27  "HWA_CLF_Target_1_ID_K2"
  Delay6/1 -> Data Type Conversion4/1
  Delay7/1 -> Data Type Conversion3/1
  Data Type Conversion3/1 -> Bus Creator/29  "HWA_CLF_Target_1_MovState_K2"
  Data Type Conversion4/1 -> Bus Creator/28  "HWA_CLF_Target_1_MovState_K1"
  HWA_CLF_Target_2/13(HWA_CLF_Target_TrgMovDirFlag_6_ObserVale) -> Bus Creator1/12  "HWA_CLF_Target_2_TrgMovDirFlag_6_ObserVale"
  LM_LR_Line04_dDisStart/1 -> Bus Creator/7  "LM_LR_Line04_dDisStart"
  LM_LR_Line04_dDisEnd/1 -> Bus Creator/8  "LM_LR_Line04_dDisEnd"
  LM_LR_Line05_dDisStart/1 -> Bus Creator/9  "LM_LR_Line05_dDisStart"
  LM_LR_Line05_dDisEnd/1 -> Bus Creator/10  "LM_LR_Line05_dDisEnd"
  LM_LR_Line06_dDisStart/1 -> Bus Creator/11  "LM_LR_Line06_dDisStart"
  LM_LR_Line06_dDisEnd/1 -> Bus Creator/12  "LM_LR_Line06_dDisEnd"
  LM_LR_Line04_pC2/1 -> Bus Creator/13  "LM_LR_Line04_pC2"
  LM_LR_Line05_pC2/1 -> Bus Creator/14  "LM_LR_Line05_pC2"
  LM_LR_Line06_pC2/1 -> Bus Creator/15  "LM_LR_Line06_pC2"
  Bus Selector/24 -> HWA_CLF_Target_2/24(LM_LR_Line04_dDisStart)  "<LM_LR_Line04_dDisStart>"
  Bus Selector/25 -> HWA_CLF_Target_2/25(LM_LR_Line04_dDisEnd)  "<LM_LR_Line04_dDisEnd>"
  Bus Selector/26 -> HWA_CLF_Target_2/26(LM_LR_Line05_dDisStart)  "<LM_LR_Line05_dDisStart>"
  Bus Selector/27 -> HWA_CLF_Target_2/27(LM_LR_Line05_dDisEnd)  "<LM_LR_Line05_dDisEnd>"
  Bus Selector/28 -> HWA_CLF_Target_2/28(LM_LR_Line06_dDisStart)  "<LM_LR_Line06_dDisStart>"
  Bus Selector/29 -> HWA_CLF_Target_2/29(LM_LR_Line06_dDisEnd)  "<LM_LR_Line06_dDisEnd>"
  Bus Selector/30 -> HWA_CLF_Target_2/30(LM_LR_Line04_pC2)  "<LM_LR_Line04_pC2>"
  Bus Selector/31 -> HWA_CLF_Target_2/31(LM_LR_Line05_pC2)  "<LM_LR_Line05_pC2>"
  Bus Selector/32 -> HWA_CLF_Target_2/32(LM_LR_Line06_pC2)  "<LM_LR_Line06_pC2>"
  LM_LR_Line04_fCamValid/1 -> Bus Creator/16  "LM_LR_Line04_fCamValid"
  LM_LR_Line05_fCamValid/1 -> Bus Creator/17  "LM_LR_Line05_fCamValid"
  LM_LR_Line06_fCamValid/1 -> Bus Creator/18  "LM_LR_Line06_fCamValid"
  Bus Selector/33 -> HWA_CLF_Target_2/33(LM_LR_Line04_fCamValid)  "<LM_LR_Line04_fCamValid>"
  Bus Selector/34 -> HWA_CLF_Target_2/34(LM_LR_Line05_fCamValid)  "<LM_LR_Line05_fCamValid>"
  Bus Selector/35 -> HWA_CLF_Target_2/35(LM_LR_Line06_fCamValid)  "<LM_LR_Line06_fCamValid>"
  HWA_CLF_Target_2/18(HWA_CLF_Target_DyConfirm_5_OverlapConfirm_ObserVale) -> Bus Creator1/17  "HWA_CLF_Target_2_DyConfirm_5_OverlapConfirm_ObserVale"
  HWA_CLF_Target_2/19(HWA_CLF_Target_DyConfirm_ALL_6_ObserVale) -> Bus Creator1/18  "HWA_CLF_Target_2_DyConfirm_ALL_6_ObserVale"
  LM_LR_Line04_pC0/1 -> Bus Creator/19  "LM_LR_Line04_pC0"
  LM_RL_Line04_pC0/1 -> Bus Creator/20  "LM_RL_Line04_pC0"
  Bus Selector/36 -> HWA_CLF_Target_2/36(LM_LR_Line04_pC0)  "<LM_LR_Line04_pC0>"
  Bus Selector/37 -> HWA_CLF_Target_2/37(LM_RL_Line04_pC0)  "<LM_RL_Line04_pC0>"
  Selector1/1 -> Delay/1, Delay1/1
  Constant1/1 -> Selector4/2, Selector3/2
  Constant/1 -> Selector1/2, Selector2/2
  TOS_HWA_Target_MovState_K1/1 -> Selector2/1
  TOS_HWA_Target_ID_K2/1 -> Selector3/1
  TOS_HWA_Target_MovState_K2/1 -> Selector4/1
  Bus Selector1/37 -> HWA_CLF_Target_1/37(LM_RL_Line04_pC0)  "<LM_RL_Line04_pC0>"
  Bus Selector1/36 -> HWA_CLF_Target_1/36(LM_LR_Line04_pC0)  "<LM_LR_Line04_pC0>"
  HWA_CLF_Target_1/19(HWA_CLF_Target_DyConfirm_ALL_6_ObserVale) -> Bus Creator2/18  "HWA_CLF_Target_1_DyConfirm_ALL_6_ObserVale"
  HWA_CLF_Target_1/18(HWA_CLF_Target_DyConfirm_5_OverlapConfirm_ObserVale) -> Bus Creator2/17  "HWA_CLF_Target_1_DyConfirm_5_OverlapConfirm_ObserVale"
  Bus Selector1/35 -> HWA_CLF_Target_1/35(LM_LR_Line06_fCamValid)  "<LM_LR_Line06_fCamValid>"
  Bus Selector1/34 -> HWA_CLF_Target_1/34(LM_LR_Line05_fCamValid)  "<LM_LR_Line05_fCamValid>"
  Bus Selector1/33 -> HWA_CLF_Target_1/33(LM_LR_Line04_fCamValid)  "<LM_LR_Line04_fCamValid>"
  Bus Selector1/32 -> HWA_CLF_Target_1/32(LM_LR_Line06_pC2)  "<LM_LR_Line06_pC2>"
  Bus Selector1/31 -> HWA_CLF_Target_1/31(LM_LR_Line05_pC2)  "<LM_LR_Line05_pC2>"
  Bus Selector1/30 -> HWA_CLF_Target_1/30(LM_LR_Line04_pC2)  "<LM_LR_Line04_pC2>"
  Bus Selector1/29 -> HWA_CLF_Target_1/29(LM_LR_Line06_dDisEnd)  "<LM_LR_Line06_dDisEnd>"
  Bus Selector1/28 -> HWA_CLF_Target_1/28(LM_LR_Line06_dDisStart)  "<LM_LR_Line06_dDisStart>"
  Bus Selector1/27 -> HWA_CLF_Target_1/27(LM_LR_Line05_dDisEnd)  "<LM_LR_Line05_dDisEnd>"
  Bus Selector1/26 -> HWA_CLF_Target_1/26(LM_LR_Line05_dDisStart)  "<LM_LR_Line05_dDisStart>"
  Bus Selector1/25 -> HWA_CLF_Target_1/25(LM_LR_Line04_dDisEnd)  "<LM_LR_Line04_dDisEnd>"
  Bus Selector1/24 -> HWA_CLF_Target_1/24(LM_LR_Line04_dDisStart)  "<LM_LR_Line04_dDisStart>"
  HWA_CLF_Target_1/13(HWA_CLF_Target_TrgMovDirFlag_6_ObserVale) -> Bus Creator2/12  "HWA_CLF_Target_1_TrgMovDirFlag_6_ObserVale"
  HWA_CLF_Target_1/16(HWA_CLF_Target_DyConfirm_3_ObserVale) -> Bus Creator2/15  "HWA_CLF_Target_1_DyConfirm_3_ObserVale"
  HWA_CLF_Target_1/15(HWA_CLF_Target_DyConfirm_2_ObserVale) -> Bus Creator2/14  "HWA_CLF_Target_1_DyConfirm_2_ObserVale"
  HWA_CLF_Target_1/14(HWA_CLF_Target_DyConfirm_1_ObserVale) -> Bus Creator2/13  "HWA_CLF_Target_1_DyConfirm_1_ObserVale"
  HWA_CLF_Target_1/12(HWA_CLF_Target_TrgMovDirFlag_5_ObserVale) -> Bus Creator2/11  "HWA_CLF_Target_1_TrgMovDirFlag_5_ObserVale"
  HWA_CLF_Target_1/11(HWA_CLF_Target_TrgMovDirFlag_4_ObserVale) -> Bus Creator2/10  "HWA_CLF_Target_1_TrgMovDirFlag_4_ObserVale"
  HWA_CLF_Target_1/10(HWA_CLF_Target_TrgMovDirFlag_3_ObserVale) -> Bus Creator2/9  "HWA_CLF_Target_1_TrgMovDirFlag_3_ObserVale"
  HWA_CLF_Target_1/9(HWA_CLF_Target_TrgMovDirFlag_2_ObserVale) -> Bus Creator2/8  "HWA_CLF_Target_1_TrgMovDirFlag_2_ObserVale"
  HWA_CLF_Target_1/8(HWA_CLF_Target_TrgMovDirFlag_1_ObserVale) -> Bus Creator2/7  "HWA_CLF_Target_1_TrgMovDirFlag_1_ObserVale"
  Bus Selector1/23 -> HWA_CLF_Target_1/23(HWA_CLF_Target_MovState_K2)  "<HWA_CLF_Target_1_MovState_K2>"
  Bus Selector1/22 -> HWA_CLF_Target_1/22(HWA_CLF_Target_MovState_K1)  "<HWA_CLF_Target_1_MovState_K1>"
  Bus Selector1/21 -> HWA_CLF_Target_1/21(HWA_CLF_Target_ID_K2)  "<HWA_CLF_Target_1_ID_K2>"
  Bus Selector1/20 -> HWA_CLF_Target_1/20(HWA_CLF_Target_ID_K1)  "<HWA_CLF_Target_1_ID_K1>"
  HWA_CLF_Target_1/17(HWA_CLF_Target_DyConfirm_4_OverlapRatio_ObserVale) -> Bus Creator2/16  "HWA_CLF_Target_1_DyConfirm_4_OverlapRatio_ObserVale"
  Bus Selector1/19 -> HWA_CLF_Target_1/19(PIL_OverlapRatio)  "<PIL_OverlapRatio>"
  Bus Selector1/18 -> HWA_CLF_Target_1/18(SteerWheelAng)  "<SteerWheelAng>"
  Bus Selector1/17 -> HWA_CLF_Target_1/17(VIE_EgoVelocity)  "<VIE_EgoVelocity>"
  Bus Selector1/16 -> HWA_CLF_Target_1/16(Object_VY)  "<Object_VY>"
  Bus Selector1/15 -> HWA_CLF_Target_1/15(Object_VX)  "<Object_VX>"
  Bus Selector1/14 -> HWA_CLF_Target_1/14(PP_ObjFusType_FC_Confirm)  "<PP_ObjFusType_FC_Confirm>"
  Bus Selector1/13 -> HWA_CLF_Target_1/13(PP_ObjFusType_FR_Confirm)  "<PP_ObjFusType_FR_Confirm>"
  Bus Selector1/12 -> HWA_CLF_Target_1/12(PP_ObjFusType_FC_FR_Confirm)  "<PP_ObjFusType_FC_FR_Confirm>"
  Bus Selector1/1 -> HWA_CLF_Target_1/1(HWA_CLF_Trg_1_Index)  "<TOS_HWA_CurrentLane_ObjIndex>"
  Bus Creator2/1 -> Terminator1/1  "HWA_CLF_Target_1_ObserVale"
  HWA_CLF_Target_1/7(HWA_CLF_Target_DyConfirm_ObserVale) -> Bus Creator2/6  "HWA_CLF_Target_1_DyConfirm_ObserVale"
  Bus Selector1/11 -> HWA_CLF_Target_1/11(Object_DY)  "<Object_DY>"
  Bus Selector1/6 -> HWA_CLF_Target_1/6(Object_HeadingAngle)  "<Object_HeadingAngle>"
  Bus Selector1/5 -> HWA_CLF_Target_1/5(PP_ObjMovingDirSignalProcessing)  "<PP_ObjMovingDirSignalProcessing>"
  HWA_CLF_Target_1/6(HWA_CLF_Target_ObstacleProb_ObserVale) -> Bus Creator2/5  "HWA_CLF_Target_1_ObstacleProb_ObserVale"
  Bus Selector1/10 -> HWA_CLF_Target_1/10(Object_ObstacleProb)  "<Object_ObstacleProb>"
  HWA_CLF_Target_1/5(HWA_CLF_Target_ObjType_ObserVale) -> Bus Creator2/4  "HWA_CLF_Target_1_ObjType_ObserVale"
  HWA_CLF_Target_1/4(HWA_CLF_Target_TargetDxConfirm_ObserVale) -> Bus Creator2/3  "HWA_CLF_Target_1_TargetDxConfirm_ObserVale"
  HWA_CLF_Target_1/3(HWA_CLF_Target_TrgMovDir_ObserVale) -> Bus Creator2/2  "HWA_CLF_Target_1_TrgMovDir_ObserVale"
  HWA_CLF_Target_1/2(HWA_CLF_Target_FusionType_ObserVale) -> Bus Creator2/1  "HWA_CLF_Target_1_FusionType_ObserVale"
  Bus Selector1/2 -> HWA_CLF_Target_1/2(Object_ID)  "<Object_ID>"
  Bus Selector1/9 -> HWA_CLF_Target_1/9(Object_Type)  "<Object_Type>"
  Bus Selector1/8 -> HWA_CLF_Target_1/8(TOS_TLJ_SameLaneConfirm_Flag)  "<TOS_TLJ_SameLaneConfirm_Flag>"
  Bus Selector1/7 -> HWA_CLF_Target_1/7(Object_DX)  "<Object_DX>"
  HWA_CLF_Target_1/1(HWA_CLF_Target_1_Index) -> [HWA_CLF_Target_1_Index], HWA_CLF_Target_1_Index/1  "HWA_CLF_Target_1_Index"
  Bus Selector1/4 -> HWA_CLF_Target_1/4(object_MovingState)  "<Object_MovingState>"
  Bus Selector1/3 -> HWA_CLF_Target_1/3(Object_Fus_Type)  "<Object_Fus_Type>"
  Bus Selector2/13 -> HWA_CLF_Target_3/13(PP_ObjFusType_FR_Confirm)  "<PP_ObjFusType_FR_Confirm>"
  Bus Selector2/11 -> HWA_CLF_Target_3/11(Object_HeadingAngle)  "<Object_HeadingAngle>"
  Bus Selector2/4 -> HWA_CLF_Target_3/4(Object_VY)  "<Object_VY>"
  Bus Selector2/3 -> HWA_CLF_Target_3/3(Object_VX)  "<Object_VX>"
  Bus Selector2/12 -> HWA_CLF_Target_3/12(PP_ObjFusType_FC_FR_Confirm)  "<PP_ObjFusType_FC_FR_Confirm>"
  Bus Selector2/5 -> HWA_CLF_Target_3/5(Object_Type)  "<Object_Type>"
  Bus Selector2/1 -> HWA_CLF_Target_3/1(HWA_CLF_Target_3)  "<TOS_HWA_CurrentLane_ObjIndex>"
  Bus Creator/1 -> Bus Selector2/1, Bus Selector/1, Bus Selector1/1
  Bus Selector2/14 -> HWA_CLF_Target_3/14(PP_ObjFusType_FC_Confirm)  "<PP_ObjFusType_FC_Confirm>"
  Bus Selector2/8 -> HWA_CLF_Target_3/8(Object_DX)  "<Object_DX>"
  Bus Selector2/2 -> HWA_CLF_Target_3/2(PP_ObjMovingDirSignalProcessing)  "<PP_ObjMovingDirSignalProcessing>"
  Bus Selector2/6 -> HWA_CLF_Target_3/6(Object_MovingState)  "<Object_MovingState>"
  Bus Selector2/15 -> HWA_CLF_Target_3/15(VIE_EgoVelocity)  "<VIE_EgoVelocity>"
  Bus Selector2/10 -> HWA_CLF_Target_3/10(Object_Fus_Type)  "<Object_Fus_Type>"
  Bus Selector2/9 -> HWA_CLF_Target_3/9(Object_DY)  "<Object_DY>"
  Bus Selector2/7 -> HWA_CLF_Target_3/7(TOS_TLJ_SameLaneConfirm_Flag)  "<TOS_TLJ_SameLaneConfirm_Flag>"
  HWA_CLF_Target_3/1(HWA_CLR_Target_3_Index) -> [HWA_CLR_Target_3_Index], HWA_CLR_Target_3_Index/1  "HWA_CLR_Target_3_Index"
  HWA_CLF_Target_3/2(HWA_CLR_Target_3_MovState_ObserVale) -> Bus Creator3/1  "HWA_CLR_Target_3_MovState_ObserVale"
  HWA_CLF_Target_3/3(HWA_CLR_Target_3_ObjType_ObserVale) -> Bus Creator3/2  "HWA_CLR_Target_3_ObjType_ObserVale"
  HWA_CLF_Target_3/4(HWA_CLR_Target_3_InCurrentLane_Flag_ObserVale) -> Bus Creator3/3  "HWA_CLR_Target_3_InCurrentLane_Flag_ObserVale"
  HWA_CLF_Target_3/5(HWA_CLR_Target_3_TargetMovingDir_ObserVale) -> Bus Creator3/4
  HWA_CLF_Target_3/6(HWA_CLR_Target_3_DyConfirm_ObserVale) -> Bus Creator3/5
  Bus Creator3/1 -> Terminator2/1
  [HWA_CLF_Target_1_Index] -> Subsystem/1(HWA_CLF_Target_1_Index)
  [HWA_CLF_Target_2_Index] -> Subsystem/2(HWA_CLF_Target_2_Index)
  [HWA_CLR_Target_3_Index] -> Subsystem/3(HWA_CLR_Target_3_Index)
  Subsystem/1(Out1) -> TargetInCurrentLane_b/1
